simulink model "Myran"  (R2021b)
settings: Solver=VariableStepAuto  StartTime=0.0  StopTime=10.0  RelTol=1e-3
settings Model: Creator=mrcha  LastModifiedBy=mrcha

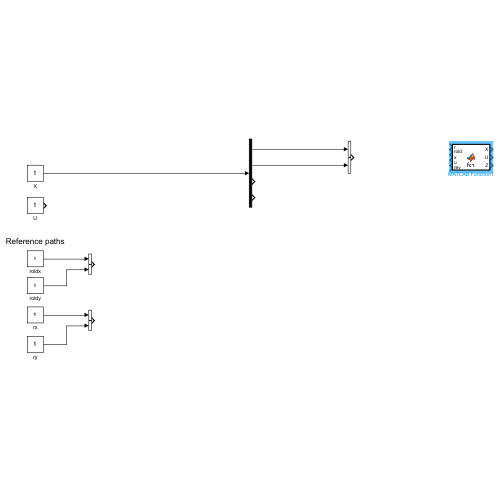
[thumbnail: Simulink's stored preview of the top-level diagram]
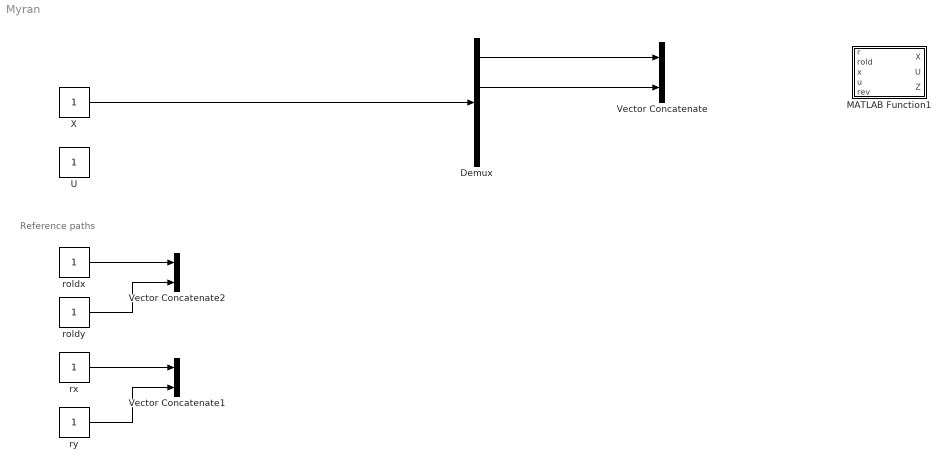
== system Myran ==
  note: Reference paths
  Demux : Demux
  MATLAB Function1 : MATLAB Function  TreatAsAtomicUnit=on
  U : Constant
  Vector Concatenate : Concatenate
  Vector Concatenate1 : Concatenate
  Vector Concatenate2 : Concatenate
  X : Constant
  roldx : Constant
  roldy : Constant
  rx : Constant
  ry : Constant
  wires:
  Demux/1 -> Vector Concatenate/1
  Demux/2 -> Vector Concatenate/2
  ry/1 -> Vector Concatenate1/2
  rx/1 -> Vector Concatenate1/1
  roldx/1 -> Vector Concatenate2/1
  roldy/1 -> Vector Concatenate2/2
  X/1 -> Demux/1

== matlab function Myran/MATLAB Function1 ==
  data: r input; rold input; x input; u input; X output; U output; Z output; rev input
function [X, U, Z] = fcn(r, rold, x, u, rev)
    % Parameters and helper functions
    params = vals();
    horiz = 5;  % Prediction horizon
    dz = 2;  % Resolution in discretised space
    % Initiate variables
    %vx = [r(1), r(2), x(3), x(4)];
    vx = x;
    ux = u;
    v0 = [vx, ux];
    % Optimization functions and parameters
    A = [0,0,0,0,1,0
        0,0,0,0,-1,0
        0,0,0,0,0,1
        0,0,0,0,0,-1
        0,0,0,1,0,0
        0,0,0,-1,0,0];
    b = [30*pi/180
        30*pi/180
        1
        1
        pi/2
        pi/2];
    % Helper functions
    z = @(x)1/x(4);  % Current lethargy
    x2 = @(x) x(1) - params(1)*cos(x(3)) - params(3)*cos(x(3) - x(4));  % x-trailer
    y2 = @(x) x(2) - params(1)*sin(x(3)) - params(3)*sin(x(3) - x(4));  % y-trailer
    dR = @(x,r) (x2(x) - r(1))^2 + (y2(x) - r(2))^2;
    px = @(r,rold,rev,dz) r(1) + (-1)^rev*(params(1)+params(3))/dz*(r(1)-rold(1));
    py = @(r,rold,rev,dz) r(1) + (-1)^rev*(params(1)+params(3))/dz*(r(2)-rold(2));
    dP = @(x,r,rold,rev,dz) (x(1) - px(r,rold,rev,dz))^2 + (x(2) - py(r,rold,rev,dz))^2;
    dr = 1;
    df = 1;
    c = @(x,u,r,rold,rev,dz) [z(x) - 1
        -z(x) - 1
        dR(x,r) - dr
        dP(x,r,rold,rev,dz) - df];
    [vx, fval] = fmincon(@(U) ObjFcn(U(1:5), U(5:7), horiz, dz, rev, r, rold), v0, A, b, Aeq, beq, lb, ub, @c);
    X = vx(1:5);
    U = vx(5:7);
    Z = z(X);
end
